simulink model "PID_control"  (R2015b)
settings: Solver=VariableStepAuto  StartTime=0.0  StopTime=10  RelTol=1e-3
settings Model: Creator=maiyf  LastModifiedBy=maiyf

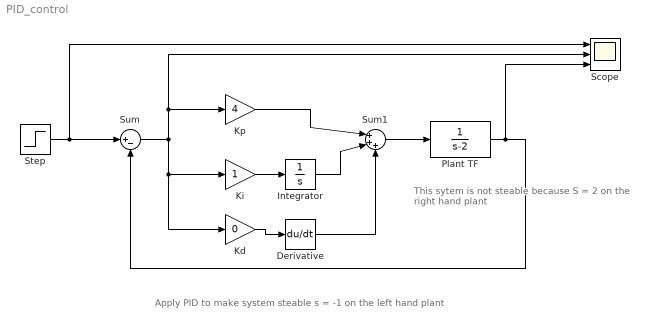
== system PID_control ==
  note: Apply PID to make system steable s = -1 on the left hand plant
  note: This sytem is not steable because S = 2 on the right hand plant
  " Plant TF" : TransferFcn  Denominator=[1 -2]
  Derivative : Derivative
  Integrator : Integrator
  Kd : Gain  Gain=0
  Ki : Gain
  Kp : Gain  Gain=4
  Scope : Scope  NumInputPorts=3
  Step : Step  Time=0.2  SampleTime=0
  Sum : Sum  Inputs=|+-
  Sum1 : Sum  Inputs=|+++
  wires:
  Step/1 -> Sum/1, Scope/1
  Sum/1 -> Ki/1, Kd/1, Scope/2, Kp/1
  " Plant TF"/1 -> Scope/3, Sum/2
  Sum1/1 -> " Plant TF"/1
  Kp/1 -> Sum1/1
  Ki/1 -> Integrator/1
  Integrator/1 -> Sum1/2
  Kd/1 -> Derivative/1
  Derivative/1 -> Sum1/3
